simulink model "EBike_Braking"  (R2019b)
settings: Solver=VariableStepAuto  StartTime=0.0  StopTime=1000  MaxStep=0.01  RelTol=1e-3
values from neighbouring files (symbols this model uses):
  A_d = 0.4    [Thesis_Ebike.m]
  Abs = 1    [Thesis_Ebike.m]
  alpha_Conductor = 0.0040    (= 0.004)    [Thesis_Ebike.m]
  Alpha_Magnet = -0.0020    (= -0.002)    [Thesis_Ebike.m]
  Bm = ((Motor_torque_constant)*(17)/(1000*2*pi/60))    (= 0.121753531465)    [Thesis_Ebike.m]
  Braking_Pressure = 100    [Thesis_Ebike.m]
  C_d = 0.9    [Thesis_Ebike.m]
  capacity = 19.5    [Thesis_Ebike.m]
  Coefficient_of_Brake_friction = 0.9    [Thesis_Ebike.m]
  Crank_Length = 0.150    (= 0.15)    [Thesis_Ebike.m]
  Cyclist_weight = 85    [Thesis_Ebike.m]
  Dynamic_Friction_Coefficient = 0.0015    [Thesis_Ebike.m]
  Effective_Radius_of_Disc = 0.16    [Thesis_Ebike.m]
  F_Rider = 100    [Thesis_Ebike.m]
  g = 9.81    [Thesis_Ebike.m]
  Internal_Resistance = 95*10^-3    (= 0.095)    [Thesis_Ebike.m]
  Jm = 10.2 *10^-3    (= 0.0102)    [Thesis_Ebike.m]
  Kb = (51.7/(1000*2*pi/60))    (= 0.493698633471)    [Thesis_Ebike.m]
  L = 0.36*10^-3    (= 0.00036)    [Thesis_Ebike.m]
  Motor_resistance = 88*10^-2    (= 0.88)    [Thesis_Ebike.m]
  Motor_torque_constant = 0.75    [Thesis_Ebike.m]
  Polarization_Capacitance = 1*10^-7    (= 1e-07)    [Thesis_Ebike.m]
  Polarization_Resistance = 95*10^-3    (= 0.095)    [Thesis_Ebike.m]
  Ref_Temp = 25    [Thesis_Ebike.m]
  Rho_air = 1.225    [Thesis_Ebike.m]
  SOC_initial = 100    [Thesis_Ebike.m]
  Static_Friction_Coefficient = 0.0015    [Thesis_Ebike.m]
  Tire_mass = 0.25    [Thesis_Ebike.m]
  Trailer_mass = 50    [Thesis_Ebike.m]
  Vehicle_mass = 25    [Thesis_Ebike.m]
  Wheel_Inertia = 0.0225    [Thesis_Ebike.m]
  Wheel_mass = 0.25    [Thesis_Ebike.m]
  Wheel_Radius = 0.3    [Thesis_Ebike.m]
undefined symbols (not defined in the file or in its folder): sigbuilder_block, V
libraries: simulink x2
(part 2 of 3)

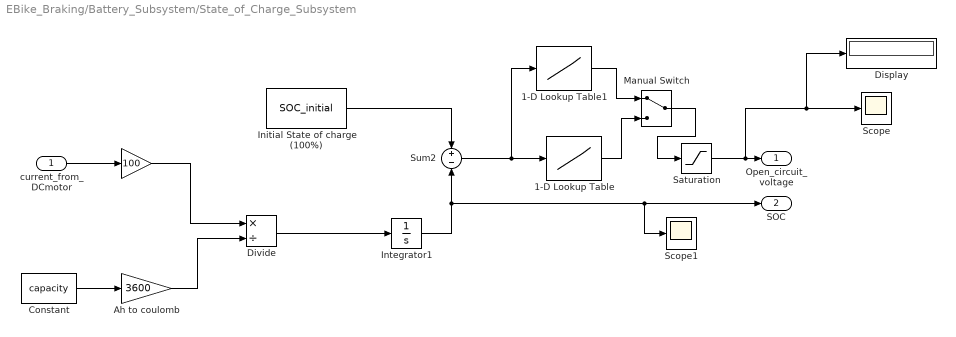
== system EBike_Braking/Battery_Subsystem/State_of_Charge_Subsystem  ==
  current_from_DCmotor : Inport
  " " : Gain  Gain=100
  1-D Lookup Table : Lookup_n-D  NumberOfTableDimensions=1  BreakpointsForDimension1=[10 12 15 20 30 45 60 75 85 95 100]  Table=|  InternalRulePriority=Speed  RndMeth=Simplest  InputSameDT=on
      | [2.75
      | 2.964
      | 3.233
      | 3.417
      | 3.65
      | 3.7
      | 3.789
      | 3.9269
      | 4.017
      | 4.147
      | 4.2
      | ]
  1-D Lookup Table1 : Lookup_n-D  NumberOfTableDimensions=1  BreakpointsForDimension1=|  Table=|  InternalRulePriority=Speed  RndMeth=Simplest  InputSameDT=on
      BreakpointsForDimension1=|
      | [-0.02
      | 0.08
      | 0.18
      | 0.28
      | 0.38
      | 0.48
      | 0.58
      | 0.68
      | 0.78
      | 0.88
      | 0.98
      | 1.08
      | 1.18
      | 1.28
      | 1.38
      | 1.48
      | 1.58
      | 1.68
      | 1.78
      | 1.88
      | 1.98
      | 2.08
      | 2.18
      | 2.28
      | 2.38
      | 2.48
      | 2.58
      | 2.68
      | 2.78
      | 2.88
      | 2.98
      | 3.08
      | 3.18
      | 3.28
      | 3.38
      | 3.48
      | 3.58
      | 3.68
      | 3.78
      | 3.88
      | 3.98
      | 4.08
      | 4.18
      | 4.28
      | 4.38
      | 4.48
      | 4.58
      | 4.68
      | 4.78
      | 4.88
      | 4.98
      | 5.08
      | 5.18
      | 5.28
      | 5.38
      | 5.48
      | 5.58
      | 5.68
      | 5.78
      | 5.88
      | 5.98
      | 6.08
      | 6.19
      | 6.29
      | 6.39
      | 6.49
      | 6.59
      | 6.69
      | 6.79
      | 6.89
      | 6.99
      | 7.09
      | 7.19
      | 7.29
      | 7.39
      | 7.49
      | 7.59
      | 7.69
      | 7.79
      | 7.89
      | 7.99
      | 8.09
      | 8.19
      | 8.29
      | 8.39
      | 8.49
      | 8.59
      | 8.69
      | 8.79
      | 8.89
      | 8.99
      | 9.09
      | 9.19
      | 9.29
      | 9.39
      | 9.49
      | 9.59
      | 9.69
      | 9.79
      | 9.89
      | 9.99
      | 10.09
      | 10.19
      | 10.29
      | 10.39
      | 10.49
      | 10.59
      | 10.69
      | 10.79
      | 10.89
      | 10.99
      | 11.09
      | 11.19
      | 11.29
      | 11.39
      | 11.49
      | 11.59
      | 11.69
      | 11.79
      | 11.89
      | 11.99
      | 12.09
      | 12.19
      | 12.29
      | 12.39
      | 12.49
      | 12.59
      | 12.69
      | 12.79
      | 12.89
      | 12.99
      | 13.09
      | 13.19
      | 13.29
      | 13.39
      | 13.49
      | 13.59
      | 13.69
      | 13.79
      | 13.89
      | 13.99
      | 14.09
      | 14.19
      | 14.29
      | 14.39
      | 14.49
      | 14.59
      | 14.69
      | 14.79
      | 14.89
      | 14.99
      | 15.09
      | 15.19
      | 15.29
      | 15.39
      | 15.49
      | 15.59
      | 15.69
      | 15.79
      | 15.89
      | 15.99
      | 16.09
      | 16.19
      | 16.29
      | 16.39
      | 16.49
      | 16.59
      | 16.69
      | 16.79
      | 16.89
      | 16.99
      | 17.09
      | 17.19
      | 17.29
      | 17.39
      | 17.49
      | 17.59
      | 17.69
      | 17.79
      | 17.89
      | 17.99
      | 18.09
      | 18.19
      | 18.29
      | 18.39
      | 18.49
      | 18.59
      | 18.69
      | 18.79
      | 18.89
      | 18.99
      | 19.09
      | 19.19
      | 19.29
      | 19.39
      | 19.49
      | 19.59
      | 19.69
      | 19.79
      | 19.89
      | 19.99
      | 20.09
      | 20.19
      | 20.29
      | 20.39
      | 20.49
      | 20.59
      | 20.69
      | 20.79
      | 20.89
      | 20.99
      | 21.09
      | 21.19
      | 21.29
      | 21.39
      | 21.49
      | 21.59
      | 21.69
      | 21.79
      | 21.89
      | 21.99
      | 22.09
      | 22.19
      | 22.29
      | 22.39
      | 22.49
      | 22.59
      | 22.69
      | 22.79
      | 22.89
      | 22.99
      | 23.09
      | 23.19
      | 23.29
      | 23.39
      | 23.49
      | 23.59
      | 23.69
      | 23.79
      | 23.89
      | 23.99
      | 24.09
      | 24.19
      | 24.29
      | 24.39
      | 24.49
      | 24.59
      | 24.69
      | 24.79
      | 24.89
      | 24.99
      | 25.09
      | 25.19
      | 25.29
      | 25.39
      | 25.49
      | 25.59
      | 25.69
      | 25.79
      | 25.89
      | 25.99
      | 26.09
      | 26.19
      | 26.29
      | 26.39
      | 26.49
      | 26.59
      | 26.69
      | 26.79
      | 26.89
      | 26.99
      | 27.09
      | 27.19
      | 27.29
      | 27.39
      | 27.49
      | 27.59
      | 27.69
      | 27.79
      | 27.89
      | 27.99
      | 28.09
      | 28.19
      | 28.29
      | 28.39
      | 28.49
      | 28.59
      | 28.69
      | 28.79
      | 28.89
      | 28.99
      | 29.09
      | 29.19
      | 29.29
      | 29.39
      | 29.49
      | 29.59
      | 29.69
      | 29.79
      | 29.89
      | 29.99
      | 30.09
      | 30.19
      | 30.29
      | 30.39
      | 30.49
      | 30.59
      | 30.69
      | 30.79
      | 30.89
      | 30.99
      | 31.09
      | 31.19
      | 31.29
      | 31.39
      | 31.49
      | 31.59
      | 31.69
      | 31.79
      | 31.89
      | 31.99
      | 32.09
      | 32.19
      | 32.29
      | 32.39
      | 32.49
      | 32.59
      | 32.69
      | 32.79
      | 32.89
      | 32.99
      | 33.09
      | 33.19
      | 33.29
      | 33.39
      | 33.49
      | 33.59
      | 33.69
      | 33.79
      | 33.89
      | 33.99
      | 34.09
      | 34.19
      | 34.29
      | 34.39
      | 34.49
      | 34.59
      | 34.69
      | 34.79
      | 34.89
      | 34.99
      | 35.09
      | 35.19
      | 35.29
      | 35.39
      | 35.49
      | 35.59
      | 35.69
      | 35.79
      | 35.89
      | 35.99
      | 36.09
      | 36.19
      | 36.29
      | 36.39
      | 36.49
      | 36.59
      | 36.69
      | 36.79
      | 36.89
      | 36.99
      | 37.09
      | 37.19
      | 37.29
      | 37.39
      | 37.49
      | 37.59
      | 37.69
      | 37.79
      | 37.89
      | 37.99
      | 38.09
      | 38.19
      | 38.29
      | 38.39
      | 38.49
      | 38.59
      | 38.69
      | 38.79
      | 38.89
      | 38.99
      | 39.09
      | 39.19
      | 39.29
      | 39.39
      | 39.49
      | 39.59
      | 39.69
      | 39.79
      | 39.89
      | 39.99
      | 40.09
      | 40.19
      | 40.29
      | 40.39
      | 40.49
      | 40.59
      | 40.69
      | 40.79
      | 40.89
      | 40.99
      | 41.09
      | 41.19
      | 41.29
      | 41.39
      | 41.49
      | 41.59
      | 41.69
      | 41.79
      | 41.89
      | 41.99
      | 42.09
      | 42.19
      | 42.29
      | 42.39
      | 42.49
      | 42.59
      | 42.69
      | 42.79
      | 42.89
      | 42.99
      | 43.09
      | 43.19
      | 43.29
      | 43.39
      | 43.49
      | 43.59
      | 43.69
      | 43.79
      | 43.89
      | 43.99
      | 44.09
      | 44.19
      | 44.29
      | 44.39
      | 44.49
      | 44.59
      | 44.69
      | 44.79
      | 44.89
      | 44.99
      | 45.09
      | 45.19
      | 45.29
      | 45.39
      | 45.49
      | 45.59
      | 45.69
      | 45.79
      | 45.89
      | 45.99
      | 46.09
      | 46.19
      | 46.29
      | 46.39
      | 46.49
      | 46.59
      | 46.69
      | 46.79
      | 46.89
      | 46.99
      | 47.09
      | 47.19
      | 47.29
      | 47.39
      | 47.49
      | 47.59
      | 47.69
      | 47.79
      | 47.89
      | 47.99
      | 48.09
      | 48.19
      | 48.29
      | 48.39
      | 48.49
      | 48.59
      | 48.69
      | 48.79
      | 48.89
      | 48.99
      | 49.09
      | 49.19
      | 49.29
      | 49.39
      | 49.49
      | 49.59
      | 49.69
      | 49.79
      | 49.89
      | 49.99
      | 50.09
      | 50.19
      | 50.29
      | 50.39
      | 50.49
      | 50.59
      | 50.69
      | 50.79
      | 50.89
      | 50.99
      | 51.09
      | 51.19
      | 51.29
      | 51.39
      | 51.49
      | 51.59
      | 51.69
      | 51.79
      | 51.89
      | 51.99
      | 52.09
      | 52.19
      | 52.29
      | 52.39
      | 52.49
      | 52.59
      | 52.69
      | 52.79
      | 52.89
      | 52.99
      | 53.09
      | 53.19
      | 53.29
      | 53.39
      | 53.49
      | 53.59
      | 53.69
      | 53.79
      | 53.89
      | 53.99
      | 54.09
      | 54.19
      | 54.29
      | 54.39
      | 54.49
      | 54.59
      | 54.69
      | 54.79
      | 54.89
      | 54.99
      | 55.09
      | 55.19
      | 55.29
      | 55.39
      | 55.49
      | 55.59
      | 55.69
      | 55.79
      | 55.89
      | 55.99
      | 56.09
      | 56.19
      | 56.29
      | 56.39
      | 56.49
      | 56.59
      | 56.69
      | 56.79
      | 56.89
      | 56.99
      | 57.09
      | 57.19
      | 57.29
      | 57.39
      | 57.49
      | 57.59
      | 57.69
      | 57.79
      | 57.89
      | 57.99
      | 58.09
      | 58.19
      | 58.29
      | 58.39
      | 58.49
      | 58.59
      | 58.69
      | 58.79
      | 58.89
      | 58.99
      | 59.09
      | 59.19
      | 59.29
      | 59.39
      | 59.49
      | 59.59
      | 59.69
      | 59.79
      | 59.89
      | 59.99
      | 60.09
      | 60.19
      | 60.29
      | 60.39
      | 60.49
      | 60.59
      | 60.69
      | 60.79
      | 60.89
      | 60.99
      | 61.09
      | 61.19
      | 61.29
      | 61.39
      | 61.49
      | 61.59
      | 61.69
      | 61.79
      | 61.89
      | 61.99
      | 62.09
      | 62.19
      | 62.29
      | 62.39
      | 62.49
      | 62.59
      | 62.69
      | 62.79
      | 62.89
      | 62.99
      | 63.09
      | 63.19
      | 63.29
      | 63.39
      | 63.49
      | 63.59
      | 63.69
      | 63.79
      | 63.89
      | 63.99
      | 64.09
      | 64.19
      | 64.29
      | 64.39
      | 64.49
      | 64.59
      | 64.69
      | 64.79
      | 64.89
      | 64.99
      | 65.09
      | 65.19
      | 65.29
      | 65.39
      | 65.49
      | 65.59
      | 65.69
      | 65.79
      | 65.89
      | 65.99
      | 66.09
      | 66.19
      | 66.29
      | 66.39
      | 66.49
      | 66.59
      | 66.69
      | 66.79
      | 66.89
      | 66.99
      | 67.09
      | 67.19
      | 67.29
      | 67.39
      | 67.49
      | 67.59
      | 67.69
      | 67.79
      | 67.89
      | 67.99
      | 68.09
      | 68.19
      | 68.29
      | 68.39
      | 68.49
      | 68.59
      | 68.69
      | 68.80
      | 68.90
      | 69.00
      | 69.10
      | 69.20
      | 69.30
      | 69.40
      | 69.50
      | 69.60
      | 69.70
      | 69.80
      | 69.90
      | 70.00
      | 70.10
      | 70.20
      | 70.30
      | 70.40
      | 70.50
      | 70.60
      | 70.70
      | 70.80
      | 70.90
      | 71.00
      | 71.10
      | 71.20
      | 71.30
      | 71.40
      | 71.50
      | 71.60
      | 71.70
      | 71.80
      | 71.90
      | 72.00
      | 72.10
      | 72.20
      | 72.30
      | 72.40
      | 72.50
      | 72.60
      | 72.70
      | 72.80
      | 72.90
      | 73.00
      | 73.10
      | 73.20
      | 73.30
      | 73.40
      | 73.50
      | 73.60
      | 73.70
      | 73.80
      | 73.90
      | 74.00
      | 74.10
      | 74.20
      | 74.30
      | 74.40
      | 74.50
      | 74.60
      | 74.70
      | 74.80
      | 74.90
      | 75.00
      | 75.10
      | 75.20
      | 75.30
      | 75.40
      | 75.50
      | 75.60
      | 75.70
      | 75.80
      | 75.90
      | 76.00
      | 76.10
      | 76.20
      | 76.30
      | 76.40
      | 76.50
      | 76.60
      | 76.70
      | 76.80
      | 76.90
      | 77.00
      | 77.10
      | 77.20
      | 77.30
      | 77.40
      | 77.50
      | 77.60
      | 77.70
      | 77.80
      | 77.90
      | 78.00
      | 78.10
      | 78.20
      | 78.30
      | 78.40
      | 78.50
      | 78.60
      | 78.70
      | 78.80
      | 78.90
      | 79.00
      | 79.10
      | 79.20
      | 79.30
      | 79.40
      | 79.50
      | 79.60
      | 79.70
      | 79.80
      | 79.90
      | 80.00
      | 80.10
      | 80.20
      | 80.30
      | 80.40
      | 80.50
      | 80.60
      | 80.70
      | 80.80
      | 80.90
      | 81.00
      | 81.10
      | 81.20
      | 81.30
      | 81.40
      | 81.50
      | 81.60
      | 81.70
      | 81.80
      | 81.90
      | 82.00
      | 82.10
      | 82.20
      | 82.30
      | 82.40
      | 82.50
      | 82.60
      | 82.70
      | 82.80
      | 82.90
      | 83.00
      | 83.10
      | 83.20
      | 83.30
      | 83.40
      | 83.50
      | 83.60
      | 83.70
      | 83.80
      | 83.90
      | 84.00
      | 84.10
      | 84.20
      | 84.30
      | 84.40
      | 84.50
      | 84.60
      | 84.70
      | 84.80
      | 84.90
      | 85.00
      | 85.10
      | 85.20
      | 85.30
      | 85.40
      | 85.50
      | 85.60
      | 85.70
      | 85.80
      | 85.90
      | 86.00
      | 86.10
      | 86.20
      | 86.30
      | 86.40
      | 86.50
      | 86.60
      | 86.70
      | 86.80
      | 86.90
      | 87.00
      | 87.10
      | 87.20
      | 87.30
      | 87.40
      | 87.50
      | 87.60
      | 87.70
      | 87.80
      | 87.90
      | 88.00
      | 88.10
      | 88.20
      | 88.30
      | 88.40
      | 88.50
      | 88.60
      | 88.70
      | 88.80
      | 88.90
      | 89.00
      | 89.10
      | 89.20
      | 89.30
      | 89.40
      | 89.50
      | 89.60
      | 89.70
      | 89.80
      | 89.90
      | 90.00
      | 90.10
      | 90.20
      | 90.30
      | 90.40
      | 90.50
      | 90.60
      | 90.70
      | 90.80
      | 90.90
      | 91.00
      | 91.10
      | 91.20
      | 91.30
      | 91.40
      | 91.50
      | 91.60
      | 91.70
      | 91.80
      | 91.90
      | 92.00
      | 92.10
      | 92.20
      | 92.30
      | 92.40
      | 92.50
      | 92.60
      | 92.70
      | 92.80
      | 92.90
      | 93.00
      | 93.10
      | 93.20
      | 93.30
      | 93.40
      | 93.50
      | 93.60
      | 93.70
      | 93.80
      | 93.90
      | 94.00
      | 94.10
      | 94.20
      | 94.30
      | 94.40
      | 94.50
      | 94.60
      | 94.70
      | 94.80
      | 94.90
      | 95.00
      | 95.10
      | 95.20
      | 95.30
      | 95.40
      | 95.50
      | 95.60
      | 95.70
      | 95.80
      | 95.90
      | 96.00
      | 96.10
      | 96.20
      | 96.30
      | 96.40
      | 96.50
      | 96.60
      | 96.70
      | 96.80
      | 96.90
      | 97.00
      | 97.10
      | 97.20
      | 97.30
      | 97.40
      | 97.50
      | 97.60
      | 97.70
      | 97.80
      | 97.90
      | 98.00
      | 98.10
      | 98.20
      | 98.30
      | 98.40
      | 98.50
      | 98.60
      | 98.70
      | 98.80
      | 98.90
      | 99.00
      | 99.10
      | 99.20
      | 99.30
      | 99.40
      | 99.50
      | 99.60
      | 99.70
      | 99.80
      | 99.90
      | ]
      Table=|
      | [26.9
      | 27.2
      | 27.4
      | 27.6
      | 27.9
      | 28.1
      | 28.3
      | 28.5
      | 28.7
      | 28.9
      | 29.1
      | 29.3
      | 29.5
      | 29.6
      | 29.8
      | 30
      | 30.1
      | 30.3
      | 30.4
      | 30.6
      | 30.7
      | 30.8
      | 31
      | 31.1
      | 31.2
      | 31.3
      | 31.4
      | 31.5
      | 31.6
      | 31.7
      | 31.8
      | 31.9
      | 32
      | 32.1
      | 32.2
      | 32.2
      | 32.3
      | 32.4
      | 32.4
      | 32.5
      | 32.6
      | 32.6
      | 32.7
      | 32.7
      | 32.8
      | 32.8
      | 32.9
      | 32.9
      | 32.9
      | 33
      | 33
      | 33.1
      | 33.1
      | 33.1
      | 33.1
      | 33.2
      | 33.2
      | 33.2
      | 33.2
      | 33.3
      | 33.3
      | 33.3
      | 33.3
      | 33.3
      | 33.3
      | 33.4
      | 33.4
      | 33.4
      | 33.4
      | 33.4
      | 33.4
      | 33.4
      | 33.5
      | 33.5
      | 33.5
      | 33.5
      | 33.5
      | 33.5
      | 33.5
      | 33.6
      | 33.6
      | 33.6
      | 33.6
      | 33.6
      | 33.6
      | 33.6
      | 33.6
      | 33.7
      | 33.7
      | 33.7
      | 33.7
      | 33.7
      | 33.7
      | 33.7
      | 33.8
      | 33.8
      | 33.8
      | 33.8
      | 33.8
      | 33.8
      | 33.8
      | 33.8
      | 33.9
      | 33.9
      | 33.9
      | 33.9
      | 33.9
      | 33.9
      | 33.9
      | 33.9
      | 33.9
      | 34
      | 34
      | 34
      | 34
      | 34
      | 34
      | 34
      | 34
      | 34
      | 34
      | 34.1
      | 34.1
      | 34.1
      | 34.1
      | 34.1
      | 34.1
      | 34.1
      | 34.1
      | 34.1
      | 34.1
      | 34.1
      | 34.2
      | 34.2
      | 34.2
      | 34.2
      | 34.2
      | 34.2
      | 34.2
      | 34.2
      | 34.2
      | 34.2
      | 34.2
      | 34.2
      | 34.3
      | 34.3
      | 34.3
      | 34.3
      | 34.3
      | 34.3
      | 34.3
      | 34.3
      | 34.3
      | 34.3
      | 34.3
      | 34.3
      | 34.3
      | 34.4
      | 34.4
      | 34.4
      | 34.4
      | 34.4
      | 34.4
      | 34.4
      | 34.4
      | 34.4
      | 34.4
      | 34.4
      | 34.4
      | 34.4
      | 34.4
      | 34.4
      | 34.5
      | 34.5
      | 34.5
      | 34.5
      | 34.5
      | 34.5
      | 34.5
      | 34.5
      | 34.5
      | 34.5
      | 34.5
      | 34.5
      | 34.5
      | 34.5
      | 34.5
      | 34.5
      | 34.6
      | 34.6
      | 34.6
      | 34.6
      | 34.6
      | 34.6
      | 34.6
      | 34.6
      | 34.6
      | 34.6
      | 34.6
      | 34.6
      | 34.6
      | 34.6
      | 34.6
      | 34.6
      | 34.6
      | 34.6
      | 34.6
      | 34.6
      | 34.7
      | 34.7
      | 34.7
      | 34.7
      | 34.7
      | 34.7
      | 34.7
      | 34.7
      | 34.7
      | 34.7
      | 34.7
      | 34.7
      | 34.7
      | 34.7
      | 34.7
      | 34.7
      | 34.7
      | 34.7
      | 34.7
      | 34.7
      | 34.7
      | 34.7
      | 34.8
      | 34.8
      | 34.8
      | 34.8
      | 34.8
      | 34.8
      | 34.8
      | 34.8
      | 34.8
      | 34.8
      | 34.8
      | 34.8
      | 34.8
      | 34.8
      | 34.8
      | 34.8
      | 34.8
      | 34.8
      | 34.8
      | 34.8
      | 34.8
      | 34.8
      | 34.8
      | 34.8
      | 34.8
      | 34.9
      | 34.9
      | 34.9
      | 34.9
      | 34.9
      | 34.9
      | 34.9
      | 34.9
      | 34.9
      | 34.9
      | 34.9
      | 34.9
      | 34.9
      | 34.9
      | 34.9
      | 34.9
      | 34.9
      | 34.9
      | 34.9
      | 34.9
      | 34.9
      | 34.9
      | 34.9
      | 34.9
      | 34.9
      | 34.9
      | 34.9
      | 35
      | 35
      | 35
      | 35
      | 35
      | 35
      | 35
      | 35
      | 35
      | 35
      | 35
      | 35
      | 35
      | 35
      | 35
      | 35
      | 35
      | 35
      | 35
      | 35
      | 35
      | 35
      | 35
      | 35
      | 35
      | 35
      | 35
      | 35
      | 35.1
      | 35.1
      | 35.1
      | 35.1
      | 35.1
      | 35.1
      | 35.1
      | 35.1
      | 35.1
      | 35.1
      | 35.1
      | 35.1
      | 35.1
      | 35.1
      | 35.1
      | 35.1
      | 35.1
      | 35.1
      | 35.1
      | 35.1
      | 35.1
      | 35.1
      | 35.1
      | 35.1
      | 35.1
      | 35.1
      | 35.1
      | 35.1
      | 35.1
      | 35.1
      | 35.1
      | 35.2
      | 35.2
      | 35.2
      | 35.2
      | 35.2
      | 35.2
      | 35.2
      | 35.2
      | 35.2
      | 35.2
      | 35.2
      | 35.2
      | 35.2
      | 35.2
      | 35.2
      | 35.2
      | 35.2
      | 35.2
      | 35.2
      | 35.2
      | 35.2
      | 35.2
      | 35.2
      | 35.2
      | 35.2
      | 35.2
      | 35.2
      | 35.2
      | 35.2
      | 35.2
      | 35.3
      | 35.3
      | 35.3
      | 35.3
      | 35.3
      | 35.3
      | 35.3
      | 35.3
      | 35.3
      | 35.3
      | 35.3
      | 35.3
      | 35.3
      | 35.3
      | 35.3
      | 35.3
      | 35.3
      | 35.3
      | 35.3
      | 35.3
      | 35.3
      | 35.3
      | 35.3
      | 35.3
      | 35.3
      | 35.3
      | 35.3
      | 35.3
      | 35.4
      | 35.4
      | 35.4
      | 35.4
      | 35.4
      | 35.4
      | 35.4
      | 35.4
      | 35.4
      | 35.4
      | 35.4
      | 35.4
      | 35.4
      | 35.4
      | 35.4
      | 35.4
      | 35.4
      | 35.4
      | 35.4
      | 35.4
      | 35.4
      | 35.4
      | 35.4
      | 35.4
      | 35.4
      | 35.4
      | 35.5
      | 35.5
      | 35.5
      | 35.5
      | 35.5
      | 35.5
      | 35.5
      | 35.5
      | 35.5
      | 35.5
      | 35.5
      | 35.5
      | 35.5
      | 35.5
      | 35.5
      | 35.5
      | 35.5
      | 35.5
      | 35.5
      | 35.5
      | 35.5
      | 35.5
      | 35.5
      | 35.6
      | 35.6
      | 35.6
      | 35.6
      | 35.6
      | 35.6
      | 35.6
      | 35.6
      | 35.6
      | 35.6
      | 35.6
      | 35.6
      | 35.6
      | 35.6
      | 35.6
      | 35.6
      | 35.6
      | 35.6
      | 35.6
      | 35.6
      | 35.6
      | 35.6
      | 35.6
      | 35.7
      | 35.7
      | 35.7
      | 35.7
      | 35.7
      | 35.7
      | 35.7
      | 35.7
      | 35.7
      | 35.7
      | 35.7
      | 35.7
      | 35.7
      | 35.7
      | 35.7
      | 35.7
      | 35.7
      | 35.7
      | 35.7
      | 35.7
      | 35.8
      | 35.8
      | 35.8
      | 35.8
      | 35.8
      | 35.8
      | 35.8
      | 35.8
      | 35.8
      | 35.8
      | 35.8
      | 35.8
      | 35.8
      | 35.8
      | 35.8
      | 35.8
      | 35.8
      | 35.8
      | 35.8
      | 35.9
      | 35.9
      | 35.9
      | 35.9
      | 35.9
      | 35.9
      | 35.9
      | 35.9
      | 35.9
      | 35.9
      | 35.9
      | 35.9
      | 35.9
      | 35.9
      | 35.9
      | 35.9
      | 35.9
      | 35.9
      | 36
      | 36
      | 36
      | 36
      | 36
      | 36
      | 36
      | 36
      | 36
      | 36
      | 36
      | 36
      | 36
      | 36
      | 36
      | 36
      | 36
      | 36.1
      | 36.1
      | 36.1
      | 36.1
      | 36.1
      | 36.1
      | 36.1
      | 36.1
      | 36.1
      | 36.1
      | 36.1
      | 36.1
      | 36.1
      | 36.1
      | 36.1
      | 36.1
      | 36.2
      | 36.2
      | 36.2
      | 36.2
      | 36.2
      | 36.2
      | 36.2
      | 36.2
      | 36.2
      | 36.2
      | 36.2
      | 36.2
      | 36.2
      | 36.2
      | 36.3
      | 36.3
      | 36.3
      | 36.3
      | 36.3
      | 36.3
      | 36.3
      | 36.3
      | 36.3
      | 36.3
      | 36.3
      | 36.3
      | 36.3
      | 36.4
      | 36.4
      | 36.4
      | 36.4
      | 36.4
      | 36.4
      | 36.4
      | 36.4
      | 36.4
      | 36.4
      | 36.4
      | 36.4
      | 36.4
      | 36.5
      | 36.5
      | 36.5
      | 36.5
      | 36.5
      | 36.5
      | 36.5
      | 36.5
      | 36.5
      | 36.5
      | 36.5
      | 36.5
      | 36.6
      | 36.6
      | 36.6
      | 36.6
      | 36.6
      | 36.6
      | 36.6
      | 36.6
      | 36.6
      | 36.6
      | 36.6
      | 36.6
      | 36.7
      | 36.7
      | 36.7
      | 36.7
      | 36.7
      | 36.7
      | 36.7
      | 36.7
      | 36.7
      | 36.7
      | 36.7
      | 36.8
      | 36.8
      | 36.8
      | 36.8
      | 36.8
      | 36.8
      | 36.8
      | 36.8
      | 36.8
      | 36.8
      | 36.9
      | 36.9
      | 36.9
      | 36.9
      | 36.9
      | 36.9
      | 36.9
      | 36.9
      | 36.9
      | 36.9
      | 36.9
      | 37
      | 37
      | 37
      | 37
      | 37
      | 37
      | 37
      | 37
      | 37
      | 37
      | 37.1
      | 37.1
      | 37.1
      | 37.1
      | 37.1
      | 37.1
      | 37.1
      | 37.1
      | 37.1
      | 37.1
      | 37.2
      | 37.2
      | 37.2
      | 37.2
      | 37.2
      | 37.2
      | 37.2
      | 37.2
      | 37.2
      | 37.2
      | 37.3
      | 37.3
      | 37.3
      | 37.3
      | 37.3
      | 37.3
      | 37.3
      | 37.3
      | 37.3
      | 37.4
      | 37.4
      | 37.4
      | 37.4
      | 37.4
      | 37.4
      | 37.4
      | 37.4
      | 37.4
      | 37.4
      | 37.5
      | 37.5
      | 37.5
      | 37.5
      | 37.5
      | 37.5
      | 37.5
      | 37.5
      | 37.5
      | 37.6
      | 37.6
      | 37.6
      | 37.6
      | 37.6
      | 37.6
      | 37.6
      | 37.6
      | 37.6
      | 37.7
      | 37.7
      | 37.7
      | 37.7
      | 37.7
      | 37.7
      | 37.7
      | 37.7
      | 37.7
      | 37.8
      | 37.8
      | 37.8
      | 37.8
      | 37.8
      | 37.8
      | 37.8
      | 37.8
      | 37.8
      | 37.8
      | 37.9
      | 37.9
      | 37.9
      | 37.9
      | 37.9
      | 37.9
      | 37.9
      | 37.9
      | 37.9
      | 38
      | 38
      | 38
      | 38
      | 38
      | 38
      | 38
      | 38
      | 38
      | 38
      | 38.1
      | 38.1
      | 38.1
      | 38.1
      | 38.1
      | 38.1
      | 38.1
      | 38.1
      | 38.1
      | 38.2
      | 38.2
      | 38.2
      | 38.2
      | 38.2
      | 38.2
      | 38.2
      | 38.2
      | 38.3
      | 38.3
      | 38.3
      | 38.3
      | 38.3
      | 38.3
      | 38.3
      | 38.3
      | 38.3
      | 38.4
      | 38.4
      | 38.4
      | 38.4
      | 38.4
      | 38.4
      | 38.4
      | 38.4
      | 38.5
      | 38.5
      | 38.5
      | 38.5
      | 38.5
      | 38.5
      | 38.5
      | 38.5
      | 38.5
      | 38.6
      | 38.6
      | 38.6
      | 38.6
      | 38.6
      | 38.6
      | 38.6
      | 38.6
      | 38.7
      | 38.7
      | 38.7
      | 38.7
      | 38.7
      | 38.7
      | 38.7
      | 38.7
      | 38.7
      | 38.8
      | 38.8
      | 38.8
      | 38.8
      | 38.8
      | 38.8
      | 38.8
      | 38.8
      | 38.9
      | 38.9
      | 38.9
      | 38.9
      | 38.9
      | 38.9
      | 38.9
      | 38.9
      | 39
      | 39
      | 39
      | 39
      | 39
      | 39
      | 39
      | 39
      | 39.1
      | 39.1
      | 39.1
      | 39.1
      | 39.1
      | 39.1
      | 39.1
      | 39.1
      | 39.2
      | 39.2
      | 39.2
      | 39.2
      | 39.2
      | 39.2
      | 39.2
      | 39.2
      | 39.3
      | 39.3
      | 39.3
      | 39.3
      | 39.3
      | 39.3
      | 39.3
      | 39.3
      | 39.4
      | 39.4
      | 39.4
      | 39.4
      | 39.4
      | 39.4
      | 39.4
      | 39.4
      | 39.5
      | 39.5
      | 39.5
      | 39.5
      | 39.5
      | 39.5
      | 39.5
      | 39.5
      | 39.6
      | 39.6
      | 39.6
      | 39.6
      | 39.6
      | 39.6
      | 39.6
      | 39.6
      | 39.7
      | 39.7
      | 39.7
      | 39.7
      | 39.7
      | 39.7
      | 39.7
      | 39.7
      | 39.8
      | 39.8
      | 39.8
      | 39.8
      | 39.8
      | 39.8
      | 39.8
      | 39.9
      | 39.9
      | 39.9
      | 39.9
      | 39.9
      | 39.9
      | 39.9
      | 39.9
      | 40
      | 40
      | 40
      | 40
      | 40
      | 40
      | 40
      | 40.1
      | 40.1
      | 40.1
      | 40.1
      | 40.1
      | 40.1
      | 40.1
      | 40.1
      | 40.2
      | 40.2
      | 40.2
      | 40.2
      | 40.2
      | 40.2
      | 40.2
      | 40.3
      | 40.3
      | 40.3
      | 40.3
      | 40.3
      | 40.3
      | 40.3
      | 40.4
      | 40.4
      | 40.4
      | 40.4
      | 40.4
      | 40.4
      | 40.4
      | 40.5
      | 40.5
      | 40.5
      | 40.5
      | 40.5
      | 40.5
      | 40.5
      | 40.6
      | 40.6
      | 40.6
      | 40.6
      | 40.6
      | 40.6
      | 40.6
      | 40.7
      | 40.7
      | 40.7
      | 40.7
      | 40.7
      | 40.7
      | 40.8
      | 40.8
      | 40.8
      | 40.8
      | 40.8
      | 40.8
      | 40.8
      | 40.9
      | 40.9
      | 40.9
      | 40.9
      | 40.9
      | 40.9
      | 41
      | 41
      | 41
      | 41
      | 41
      | 41
      | 41
      | 41.1
      | 41.1
      | 41.1
      | 41.1
      | 41.1
      | 41.1
      | 41.2
      | ]
  Ah to coulomb : Gain  Gain=3600
  Constant : Constant  Value=capacity  SampleTime=-1
  Display : Display
  Divide : Product  Inputs=*/
  Initial State of charge (100%) : Constant  Value=SOC_initial  SampleTime=-1
  Integrator1 : Integrator  UpperSaturationLimit=100  LowerSaturationLimit=0
  Manual Switch : ManualSwitch
  Saturation : Saturate  UpperLimit=inf  LowerLimit=0
  Scope : Scope
  Scope1 : Scope
  Sum2 : Sum  Inputs=+|-
  Open_circuit_voltage : Outport  VectorParamsAs1DForOutWhenUnconnected=off
  SOC : Outport  Port=2  VectorParamsAs1DForOutWhenUnconnected=off
  wires:
  Integrator1/1 -> Scope1/1, SOC/1, Sum2/2
  Initial State of charge (100%)/1 -> Sum2/1
  Divide/1 -> Integrator1/1
  Saturation/1 -> Display/1, Scope/1, Open_circuit_voltage/1
  Sum2/1 -> 1-D Lookup Table/1, 1-D Lookup Table1/1
  Ah to coulomb/1 -> Divide/2
  current_from_DCmotor/1 -> " "/1
  Constant/1 -> Ah to coulomb/1
  " "/1 -> Divide/1
  1-D Lookup Table1/1 -> Manual Switch/1
  Manual Switch/1 -> Saturation/1
  1-D Lookup Table/1 -> Manual Switch/2

== system EBike_Braking/Bike_Mechanics_subsystem/Aerodynamic_Drag_subsystem ==
  Vehicle Speed (V) : Inport
  "Wind Speed (V_w) " : Inport  Port=2
  . : Constant  Value=1/2
  Air_density : Constant  Value=Rho_air
  Cross sectional area/Reference area : Constant  Value=A_d
  Drag Coeffient : Constant  Value=C_d
  Drag_force_scope : Scope
  Math Function1 : Math  Operator=square  SaturateOnIntegerOverflow=on
  Product : Product  Inputs=5
  Sum : Sum  Inputs=+-
  "Drag_Force " : Outport  VectorParamsAs1DForOutWhenUnconnected=off
  wires:
  Product/1 -> Drag_force_scope/1, "Drag_Force "/1
  ./1 -> Product/1
  Air_density/1 -> Product/2
  Drag Coeffient/1 -> Product/3
  Cross sectional area/Reference area/1 -> Product/4
  Math Function1/1 -> Product/5
  "Wind Speed (V_w) "/1 -> Sum/2
  Vehicle Speed (V)/1 -> Sum/1
  Sum/1 -> Math Function1/1

== system EBike_Braking/Bike_Mechanics_subsystem/Gradient_Resistance_subsystem ==
  Angle_of_slope : Inport
  Acceleration due to Gravity (g) m/s^2 : Constant  Value=g  SampleTime=-1
  Cos : Trigonometry
  Cyclist_weight (M) in Kg : Constant  Value=Cyclist_weight  SampleTime=-1
  Display : Display
  Gradient_resistance_scope : Scope
  Product : Product  Inputs=3
  Scope : Scope
  Sum2 : Sum
  Vehicle_mass (M) in Kg : Constant  Value=Vehicle_mass  SampleTime=-1
  Gradient_resistance : Outport  VectorParamsAs1DForOutWhenUnconnected=off
  wires:
  Product/1 -> Gradient_resistance_scope/1, Gradient_resistance/1
  Angle_of_slope/1 -> Cos/1
  Acceleration due to Gravity (g) m/s^2/1 -> Product/2
  Cos/1 -> Scope/1, Display/1, Product/3
  Sum2/1 -> Product/1
  Cyclist_weight (M) in Kg/1 -> Sum2/1
  Vehicle_mass (M) in Kg/1 -> Sum2/2

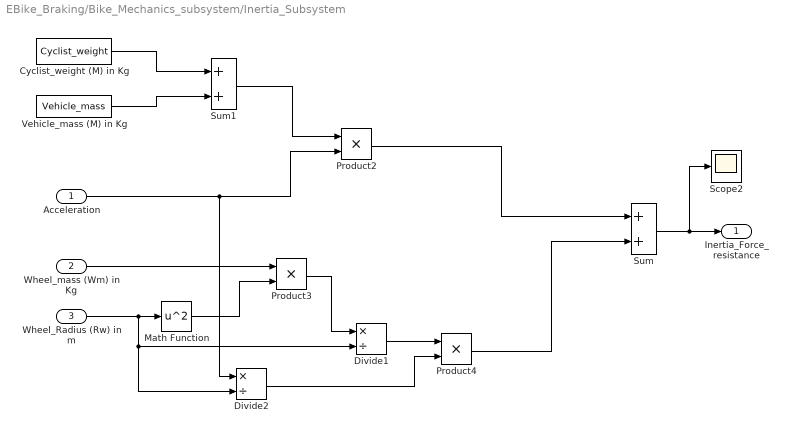
== system EBike_Braking/Bike_Mechanics_subsystem/Inertia_Subsystem ==
  Acceleration : Inport
  Wheel_mass (Wm) in Kg : Inport  Port=2
  Wheel_Radius (Rw) in m : Inport  Port=3
  Cyclist_weight (M) in Kg : Constant  Value=Cyclist_weight  SampleTime=-1
  Divide1 : Product  Inputs=*/
  Divide2 : Product  Inputs=*/
  Math Function : Math  Operator=square  SaturateOnIntegerOverflow=on
  Product2 : Product
  Product3 : Product
  Product4 : Product
  Scope2 : Scope
  Sum : Sum
  Sum1 : Sum
  Vehicle_mass (M) in Kg : Constant  Value=Vehicle_mass  SampleTime=-1
  Inertia_Force_resistance : Outport
  wires:
  Wheel_Radius (Rw) in m/1 -> Divide2/2, Divide1/2, Math Function/1
  Wheel_mass (Wm) in Kg/1 -> Product3/1
  Math Function/1 -> Product3/2
  Cyclist_weight (M) in Kg/1 -> Sum1/1
  Vehicle_mass (M) in Kg/1 -> Sum1/2
  Acceleration/1 -> Divide2/1, Product2/2
  Sum1/1 -> Product2/1
  Product3/1 -> Divide1/1
  Divide1/1 -> Product4/1
  Divide2/1 -> Product4/2
  Sum/1 -> Scope2/1, Inertia_Force_resistance/1
  Product2/1 -> Sum/1
  Product4/1 -> Sum/2

== system EBike_Braking/Bike_Mechanics_subsystem/Inertia_Subsystem1 ==
  Acceleration : Inport
  Gain : Gain
  Product2 : Product
  Scope2 : Scope
  Vehicle_mass (M) in Kg : Constant  Value=Trailer_mass  SampleTime=-1
  Trailer_force : Outport
  wires:
  Product2/1 -> Gain/1
  Vehicle_mass (M) in Kg/1 -> Product2/1
  Acceleration/1 -> Product2/2
  Gain/1 -> Scope2/1, Trailer_force/1

== system EBike_Braking/Bike_Mechanics_subsystem/Pedallic_torque_subsystem ==
  Torque : Inport
  Gear_ratio : Inport  Port=2
  Divide : Product  Inputs=*/
  Divide1 : Product  Inputs=*/
  Scope : Scope
  Scope1 : Scope
  Scope2 : Scope
  "Wheel_radius (Rw) " : Constant  Value=Wheel_Radius  SampleTime=-1
  Drive_Force : Outport  VectorParamsAs1DForOutWhenUnconnected=off
  wires:
  Gear_ratio/1 -> Divide1/2
  Divide1/1 -> Scope/1, Divide/1
  "Wheel_radius (Rw) "/1 -> Divide/2
  Divide/1 -> Scope2/1, Drive_Force/1
  Torque/1 -> Divide1/1, Scope1/1

== system EBike_Braking/Bike_Mechanics_subsystem/Rolling_Resistance_subsystem ==
  Angle_of_slope : Inport
  Acceleration_due_to_Gravity (g) m/s^2 : Constant  Value=g  SampleTime=-1
  Cos : Trigonometry  Operator=cos
  Cyclist_weight (M) in Kg : Constant  Value=Cyclist_weight  SampleTime=-1
  Dynamic_Friction_Coefficient : Constant  Value=Dynamic_Friction_Coefficient  SampleTime=-1
  Product : Product  Inputs=4
  Rolling_resistance_scope : Scope
  Static_Friction_Coefficient : Constant  Value=Static_Friction_Coefficient  SampleTime=-1
  Sum : Sum  Inputs=+|+
  Sum2 : Sum
  Vehicle_mass (M) in Kg : Constant  Value=Vehicle_mass  SampleTime=-1
  Rolling_resistance : Outport  VectorParamsAs1DForOutWhenUnconnected=off
  wires:
  Acceleration_due_to_Gravity (g) m/s^2/1 -> Product/3
  Product/1 -> Rolling_resistance/1, Rolling_resistance_scope/1
  Cos/1 -> Product/4
  Angle_of_slope/1 -> Cos/1
  Static_Friction_Coefficient/1 -> Sum/1
  Dynamic_Friction_Coefficient/1 -> Sum/2
  Sum/1 -> Product/1
  Sum2/1 -> Product/2
  Cyclist_weight (M) in Kg/1 -> Sum2/1
  Vehicle_mass (M) in Kg/1 -> Sum2/2

== system EBike_Braking/Bike_Mechanics_subsystem/Subsystem2 ==
  Slope % : Inport
  Constant : Constant  Value=pi  SampleTime=-1
  Constant1 : Constant  Value=180
  Divide : Product  Inputs=*/
  Gain : Gain  Gain=1/1
  Product : Product
  Trigonometric Function : Trigonometry  Operator=atan
  alpha : Outport  VectorParamsAs1DForOutWhenUnconnected=off
  wires:
  Gain/1 -> Trigonometric Function/1
  Slope %/1 -> Gain/1
  Trigonometric Function/1 -> Product/1
  Product/1 -> alpha/1
  Constant/1 -> Divide/1
  Constant1/1 -> Divide/2
  Divide/1 -> Product/2

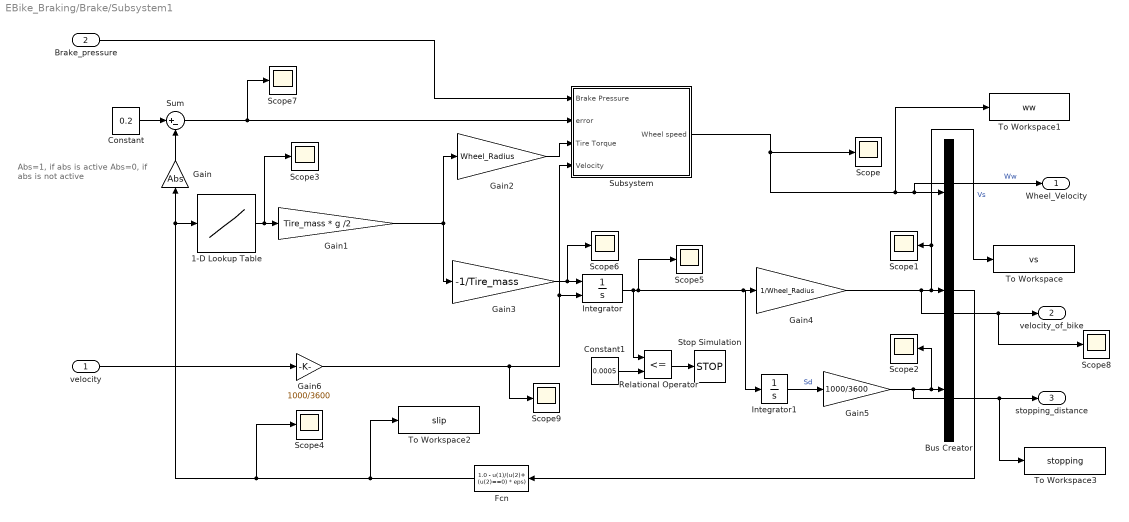
== system EBike_Braking/Brake/Subsystem1 ==
  note: Abs=1, if abs is active
      | Abs=0, if abs is not active
  velocity : Inport
  Brake_pressure : Inport  Port=2
  1-D Lookup Table : Lookup_n-D  NumberOfTableDimensions=1  BreakpointsForDimension1="[0\t0.0500000000000000\t0.100000000000000\t0.150000000000000\t0.200000000000000\t0.250000000000000\t0.300000000000000\t0.350000000000000\t0.400000000000000\t0.450000000000000\t0.500000000000000\t0.550000000000000\t0.600000000000000\t0.650000000000000\t0.700000000000000\t0.750000000000000\t0.800000000000000\t0.850000000000000\t0.900000000000000\t0.950000000000000\t1]"  Table="[0\t0.400000000000000\t0.800000000000000\t0.970000000000000\t1\t0.980000000000000\t0.960000000000000\t0.940000000000000\t0.920000000000000\t0.900000000000000\t0.880000000000000\t0.855000000000000\t0.830000000000000\t0.810000000000000\t0.790000000000000\t0.770000000000000\t0.750000000000000\t0.730000000000000\t0.720000000000000\t0.710000000000000\t0.700000000000000]"  InternalRulePriority=Speed  RndMeth=Simplest  InputSameDT=on
  Bus Creator : BusCreator  Inputs=3
  Constant : Constant  Value=0.2
  Constant1 : Constant  Value=0.0005
  Fcn : Fcn  Expr=1.0 - u(1)/(u(2)+ (u(2)==0) * eps)
  Gain : Gain  Gain=Abs
  Gain1 : Gain  Gain=Tire_mass * g /2
  Gain2 : Gain  Gain=Wheel_Radius
  Gain3 : Gain  Gain=-1/Tire_mass
  Gain4 : Gain  Gain=1/Wheel_Radius
  Gain5 : Gain  Gain=1000/3600
  Gain6 : Gain  Gain=1000/3600
  Integrator : Integrator  InitialConditionSource=external  InitialCondition=V  LimitOutput=on  UpperSaturationLimit=1000  LowerSaturationLimit=0  ZeroCross=off
  Integrator1 : Integrator
  Relational Operator : RelationalOperator  Operator=<=  OutDataTypeStr=boolean  RndMeth=Simplest
  Scope{,1..9} (10 alike) : Scope
  Stop Simulation : Stop
  Subsystem : Subsystem
  Sum : Sum  Inputs=|+-
  To Workspace : ToWorkspace  VariableName=vs  SaveFormat=Timeseries  SampleTime=-1
  To Workspace1 : ToWorkspace  VariableName=ww  SaveFormat=Timeseries  SampleTime=-1
  To Workspace2 : ToWorkspace  VariableName=slip  SaveFormat=Timeseries  SampleTime=-1
  To Workspace3 : ToWorkspace  VariableName=stopping  SaveFormat=Timeseries  SampleTime=-1
  Wheel_Velocity : Outport
  velocity_of_bike : Outport  Port=2
  stopping_distance : Outport  Port=3
  wires:
  Subsystem/1("Wheel speed ") -> Scope/1, To Workspace1/1, Wheel_Velocity/1, Bus Creator/1  "Ww"
  Integrator1/1 -> Gain5/1  "Sd"
  Sum/1 -> Subsystem/2("error "), Scope7/1
  Gain1/1 -> Gain3/1, Gain2/1
  Gain2/1 -> Subsystem/3(Tire Torque)
  Gain/1 -> Sum/2
  1-D Lookup Table/1 -> Scope3/1, Gain1/1
  Gain3/1 -> Scope6/1, Integrator/1
  Constant/1 -> Sum/1
  Gain4/1 -> To Workspace/1, Scope1/1, Bus Creator/2, Scope8/1, velocity_of_bike/1  "Vs"
  Fcn/1 -> To Workspace2/1, Scope4/1, 1-D Lookup Table/1, Gain/1
  Bus Creator/1 -> Fcn/1
  Constant1/1 -> Relational Operator/2
  Relational Operator/1 -> Stop Simulation/1
  Integrator/1 -> Integrator1/1, Gain4/1, Scope5/1, Relational Operator/1
  Gain5/1 -> To Workspace3/1, stopping_distance/1, Scope2/1, Bus Creator/3
  Gain6/1 -> Scope9/1, Subsystem/4(Velocity), Integrator/2
  Brake_pressure/1 -> Subsystem/1(Brake Pressure)
  velocity/1 -> Gain6/1

== system EBike_Braking/Controller/If Action Subsystem1 ==
  In1 : Inport
  Action Port : ActionPort  ActionPortLabel=if(u1<26)
  Gain : Gain
  Out1 : Outport
  wires:
  In1/1 -> Gain/1
  Gain/1 -> Out1/1

== system EBike_Braking/Controller/If Action Subsystem11 ==
  In1 : Inport
  Action Port : ActionPort  ActionPortLabel=if(u1 > 0)
  Gain : Gain  Gain=0
  Out1 : Outport
  wires:
  Gain/1 -> Out1/1
  In1/1 -> Gain/1

== system EBike_Braking/Controller/If Action Subsystem12 ==
  In1 : Inport
  Action Port : ActionPort  ActionPortLabel=else
  Gain : Gain
  Out1 : Outport
  wires:
  Gain/1 -> Out1/1
  In1/1 -> Gain/1

== system EBike_Braking/Controller/If Action Subsystem8 ==
  In1 : Inport
  Action Port : ActionPort  ActionPortLabel=else
  Gain : Gain  Gain=0
  Out1 : Outport
  wires:
  Gain/1 -> Out1/1
  In1/1 -> Gain/1

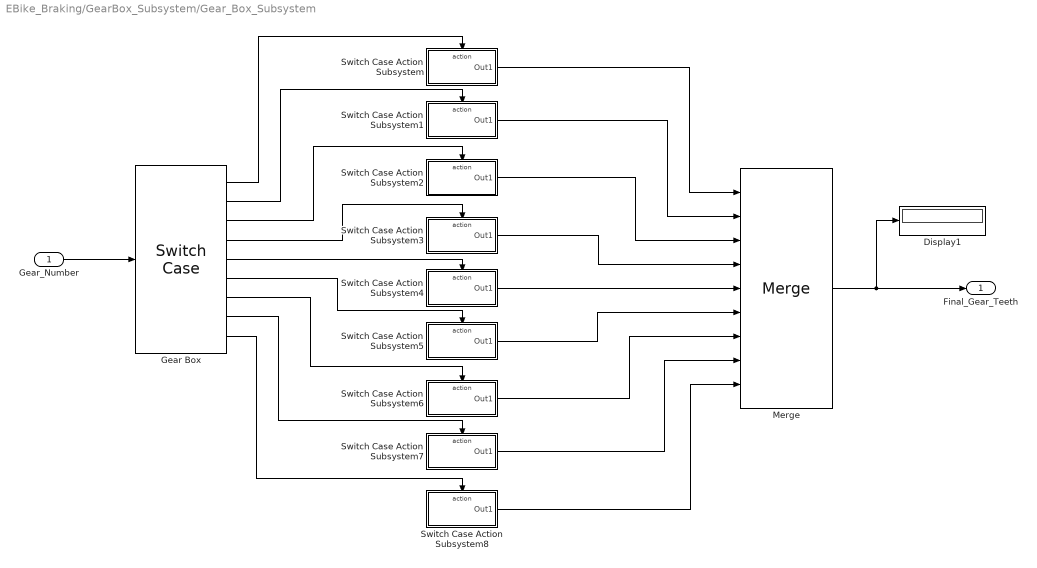
== system EBike_Braking/GearBox_Subsystem/Gear_Box_Subsystem ==
  Gear_Number : Inport
  Display1 : Display
  Gear Box : SwitchCase  CaseConditions={1,2,3,4,5,6,7,8,9}  ShowDefaultCase=off
  Merge : Merge  Inputs=9
  Switch Case Action Subsystem : Subsystem  TreatAsAtomicUnit=on
  Switch Case Action Subsystem1 : Subsystem  TreatAsAtomicUnit=on
  Switch Case Action Subsystem2 : Subsystem  TreatAsAtomicUnit=on
  Switch Case Action Subsystem3 : Subsystem  TreatAsAtomicUnit=on
  Switch Case Action Subsystem4 : Subsystem  TreatAsAtomicUnit=on
  Switch Case Action Subsystem5 : Subsystem  TreatAsAtomicUnit=on
  Switch Case Action Subsystem6 : Subsystem  TreatAsAtomicUnit=on
  Switch Case Action Subsystem7 : Subsystem  TreatAsAtomicUnit=on
  Switch Case Action Subsystem8 : Subsystem  TreatAsAtomicUnit=on
  Final_Gear_Teeth : Outport  VectorParamsAs1DForOutWhenUnconnected=off
  wires:
  Gear Box/5 -> Switch Case Action Subsystem4/Action
  Gear Box/2 -> Switch Case Action Subsystem1/Action
  Gear Box/4 -> Switch Case Action Subsystem3/Action
  Gear Box/9 -> Switch Case Action Subsystem8/Action
  Gear Box/7 -> Switch Case Action Subsystem6/Action
  Gear Box/6 -> Switch Case Action Subsystem5/Action
  Gear Box/3 -> Switch Case Action Subsystem2/Action
  Gear Box/1 -> Switch Case Action Subsystem/Action
  Merge/1 -> Display1/1, Final_Gear_Teeth/1
  Gear Box/8 -> Switch Case Action Subsystem7/Action
  Gear_Number/1 -> Gear Box/1
  Switch Case Action Subsystem8/1(Out1) -> Merge/9
  Switch Case Action Subsystem7/1(Out1) -> Merge/8
  Switch Case Action Subsystem6/1(Out1) -> Merge/7
  Switch Case Action Subsystem5/1(Out1) -> Merge/6
  Switch Case Action Subsystem4/1(Out1) -> Merge/5
  Switch Case Action Subsystem3/1(Out1) -> Merge/4
  Switch Case Action Subsystem2/1(Out1) -> Merge/3
  Switch Case Action Subsystem1/1(Out1) -> Merge/2
  Switch Case Action Subsystem/1(Out1) -> Merge/1

== system EBike_Braking/Motor_Subsystem/Magnetic_Flux_density_subsystem ==
  Ambient_temp_T : Inport
  Motor_torque_constant_at_Temp_T0 : Inport  Port=2
  Constant : Constant
  Product : Product
  Product1 : Product
  Reference_temp_T0 : Constant  Value=Ref_Temp
  Sum1 : Sum  Inputs=+-
  Sum2 : Sum
  Temperature_Coefficient : Constant  Value=Alpha_Magnet
  Motor_Torque_Constant_at_Temp_T : Outport  VectorParamsAs1DForOutWhenUnconnected=off
  wires:
  Motor_torque_constant_at_Temp_T0/1 -> Product1/1
  Product1/1 -> Motor_Torque_Constant_at_Temp_T/1
  Product/1 -> Sum2/2
  Constant/1 -> Sum2/1
  Sum2/1 -> Product1/2
  Temperature_Coefficient/1 -> Product/1
  Ambient_temp_T/1 -> Sum1/1
  Reference_temp_T0/1 -> Sum1/2
  Sum1/1 -> Product/2

== system EBike_Braking/Motor_Subsystem/Winding_resistance_Subsystem ==
  Resistance_at_Temp_T0 : Inport
  Ambient_temp_T : Inport  Port=2
  Constant : Constant
  Product : Product
  Product1 : Product
  Reference_temp_T0 : Constant  Value=Ref_Temp
  Resistance_Temperature_Coefficient : Constant  Value=alpha_Conductor
  Sum1 : Sum  Inputs=+-
  Sum2 : Sum
  Resistance_at_Temp_T : Outport  VectorParamsAs1DForOutWhenUnconnected=off
  wires:
  Sum1/1 -> Product/2
  Reference_temp_T0/1 -> Sum1/2
  Ambient_temp_T/1 -> Sum1/1
  Resistance_Temperature_Coefficient/1 -> Product/1
  Sum2/1 -> Product1/2
  Constant/1 -> Sum2/1
  Product/1 -> Sum2/2
  Product1/1 -> Resistance_at_Temp_T/1
  Resistance_at_Temp_T0/1 -> Product1/1

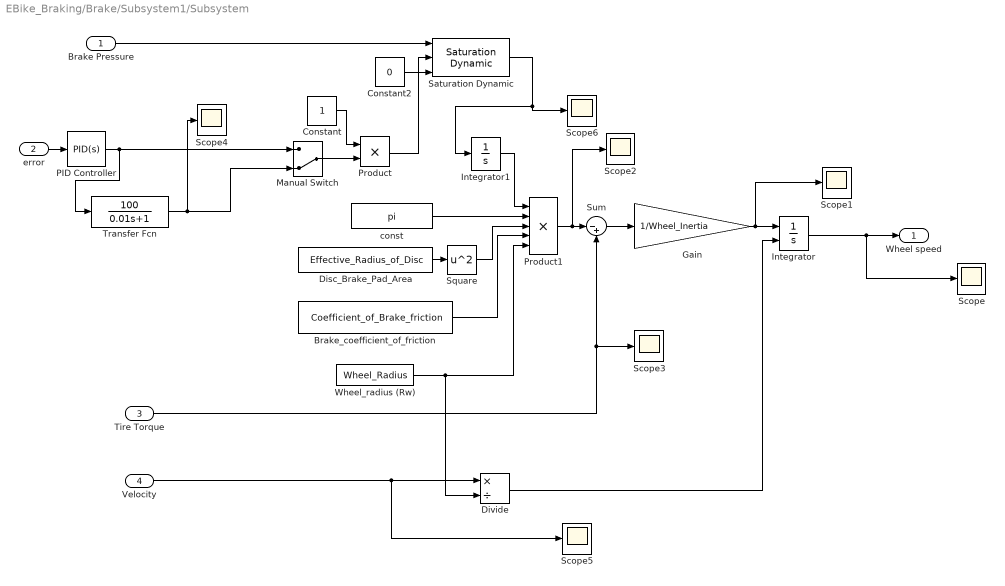
== system EBike_Braking/Brake/Subsystem1/Subsystem ==
  Brake Pressure : Inport
  "error " : Inport  Port=2
  Tire Torque : Inport  Port=3
  Velocity : Inport  Port=4
  Brake_coefficient_of_friction : Constant  Value=Coefficient_of_Brake_friction
  Constant : Constant
  Constant2 : Constant  Value=0
  Disc_Brake_Pad_Area : Constant  Value=Effective_Radius_of_Disc
  Divide : Product  Inputs=*/
  Gain : Gain  Gain=1/Wheel_Inertia
  Integrator : Integrator  InitialConditionSource=external  InitialCondition=V/Wheel_Radius  LimitOutput=on  UpperSaturationLimit=1000  LowerSaturationLimit=0
  Integrator1 : Integrator  UpperSaturationLimit=Braking_Pressure
  Manual Switch : ManualSwitch  CurrentSetting=0
  PID Controller : simulink/Continuous/PID Controller  Controller=PID  Form=Parallel  TimeDomain=Continuous-time  SampleTime=-1  IntegratorMethod=Forward Euler  FilterMethod=Forward Euler  ControllerParametersSource=internal  P=22  I=4  D=0.4  UseFilter=on  N=100  TunerSelectOption=Transfer Function Based (PID Tuner App)  InitialConditionSource=internal  InitialConditionForIntegrator=0  InitialConditionForFilter=0  DifferentiatorICPrevScaledInput=0  ExternalReset=none  TrackingMode=off  Kt=1  LimitOutput=off  UpperSaturationLimit=inf  LowerSaturationLimit=-inf  LinearizeAsGain=on  AntiWindupMode=none  Kb=1  POutMin=[]  POutMax=[]  IOutMin=[]  IOutMax=[]  DOutMin=[]  DOutMax=[]  NOutMin=[]  NOutMax=[]  SumOutMin=[]  SumOutMax=[]  SaturationOutMin=[]  SaturationOutMax=[]  PParamMin=[]  PParamMax=[]  IParamMin=[]  IParamMax=[]  DParamMin=[]  DParamMax=[]  NParamMin=[]  NParamMax=[]  KbParamMin=[]  KbParamMax=[]  KtParamMin=[]  KtParamMax=[]  KbOutMin=[]  KbOutMax=[]  KtOutMin=[]  KtOutMax=[]  IntegratorOutMin=[]  IntegratorOutMax=[]  FilterOutMin=[]  FilterOutMax=[]  SumI1OutMin=[]  SumI1OutMax=[]  SumI2OutMin=[]  SumI2OutMax=[]  SumI3OutMin=[]  SumI3OutMax=[]  SumI4OutMin=[]  SumI4OutMax=[]  SumDOutMin=[]  SumDOutMax=[]  DifferentiatorOutMin=[]  DifferentiatorOutMax=[]  FilterDiffOutCoefMin=[]  FilterDiffOutCoefMax=[]  ReciprocalOutMin=[]  ReciprocalOutMax=[]  SumDenOutMin=[]  SumDenOutMax=[]  SumNumOutMin=[]  SumNumOutMax=[]  DivideOutMin=[]  DivideOutMax=[]  IntegratorContinuousStateAttributes=''  IntegratorStateMustResolveToSignalObject=off  IntegratorRTWStateStorageClass=Auto  FilterContinuousStateAttributes=''  FilterStateMustResolveToSignalObject=off  FilterRTWStateStorageClass=Auto  ParallelPVariant=InternalParameters  IdealPVariant=Disabled  IVariant=InternalParameters  DVariant=InternalParameters  IntegratorVariant=Continuous  SatVariant=Disabled  AWVariant=Passthrough  PCopyVariant=Disabled  TRVariant=Disabled  FdbkBlocksVariant=Forward  IdealPFdbkVariant=Disabled  SatFdbkVariant=Disabled  DerivativeFilterVariant=ContFilter  NVariant=InternalParameters  NCopyVariant=Disabled  FilterICVariant=InternalICsFilter  IntegratorICVariant=InternalICs  ExternalResetVariant=Disabled  TRSumVariant=Passthrough  SumFdbkVariant=Disabled  SumVariant=Sum_PID
  Product : Product
  Product1 : Product  Inputs=5
  Saturation Dynamic : simulink/Discontinuities/Saturation Dynamic  OutMin=[]  OutMax=[]  OutDataTypeStr=Inherit: Same as second input  OutDataType=fixdt(1, 16)  OutScaling=2^-10  DoSatur=off
  Scope{,1..6} (7 alike) : Scope
  Square : Math  Operator=square  SaturateOnIntegerOverflow=on
  Sum : Sum  Inputs=|-+
  Transfer Fcn : TransferFcn  Numerator=[100]  Denominator=[0.01 1]
  "Wheel_radius (Rw) " : Constant  Value=Wheel_Radius
  "const " : Constant  Value=pi
  "Wheel speed " : Outport
  wires:
  "error "/1 -> PID Controller/1
  Constant/1 -> Product/1
  "const "/1 -> Product1/2
  Disc_Brake_Pad_Area/1 -> Square/1
  Square/1 -> Product1/3
  Brake_coefficient_of_friction/1 -> Product1/4
  Product1/1 -> Scope2/1, Sum/1
  Tire Torque/1 -> Scope3/1, Sum/2
  Sum/1 -> Gain/1
  Gain/1 -> Scope1/1, Integrator/1
  Manual Switch/1 -> Product/2
  PID Controller/1 -> Transfer Fcn/1, Manual Switch/1
  Integrator1/1 -> Product1/1
  Velocity/1 -> Scope5/1, Divide/1
  Divide/1 -> Integrator/2
  "Wheel_radius (Rw) "/1 -> Divide/2, Product1/5
  Integrator/1 -> "Wheel speed "/1, Scope/1
  Transfer Fcn/1 -> Scope4/1, Manual Switch/2
  Constant2/1 -> Saturation Dynamic/3
  Product/1 -> Saturation Dynamic/2
  Saturation Dynamic/1 -> Scope6/1, Integrator1/1
  Brake Pressure/1 -> Saturation Dynamic/1

== system EBike_Braking/GearBox_Subsystem/Gear_Box_Subsystem/Switch Case Action Subsystem ==
  Action Port : ActionPort  ActionPortLabel=case [ 1 ]:
  Constant : Constant  Value=34
  Out1 : Outport  VectorParamsAs1DForOutWhenUnconnected=off
  wires:
  Constant/1 -> Out1/1

== system EBike_Braking/GearBox_Subsystem/Gear_Box_Subsystem/Switch Case Action Subsystem1 ==
  Action Port : ActionPort  ActionPortLabel=case [ 2 ]:
  Constant : Constant  Value=30
  Out1 : Outport  VectorParamsAs1DForOutWhenUnconnected=off
  wires:
  Constant/1 -> Out1/1

== system EBike_Braking/GearBox_Subsystem/Gear_Box_Subsystem/Switch Case Action Subsystem2 ==
  Action Port : ActionPort  ActionPortLabel=case [ 3 ]:
  Constant : Constant  Value=26
  Out1 : Outport  VectorParamsAs1DForOutWhenUnconnected=off
  wires:
  Constant/1 -> Out1/1

== system EBike_Braking/GearBox_Subsystem/Gear_Box_Subsystem/Switch Case Action Subsystem3 ==
  Action Port : ActionPort  ActionPortLabel=case [ 4 ]:
  Constant : Constant  Value=23
  Out1 : Outport  VectorParamsAs1DForOutWhenUnconnected=off
  wires:
  Constant/1 -> Out1/1

== system EBike_Braking/GearBox_Subsystem/Gear_Box_Subsystem/Switch Case Action Subsystem4 ==
  Action Port : ActionPort  ActionPortLabel=case [ 5 ]:
  Constant : Constant  Value=20
  Out1 : Outport  VectorParamsAs1DForOutWhenUnconnected=off
  wires:
  Constant/1 -> Out1/1

== system EBike_Braking/GearBox_Subsystem/Gear_Box_Subsystem/Switch Case Action Subsystem5 ==
  Action Port : ActionPort  ActionPortLabel=case [ 6 ]:
  Constant : Constant  Value=17
  Out1 : Outport  VectorParamsAs1DForOutWhenUnconnected=off
  wires:
  Constant/1 -> Out1/1

== system EBike_Braking/GearBox_Subsystem/Gear_Box_Subsystem/Switch Case Action Subsystem6 ==
  Action Port : ActionPort  ActionPortLabel=case [ 7 ]:
  Constant : Constant  Value=15
  Out1 : Outport  VectorParamsAs1DForOutWhenUnconnected=off
  wires:
  Constant/1 -> Out1/1

== system EBike_Braking/GearBox_Subsystem/Gear_Box_Subsystem/Switch Case Action Subsystem7 ==
  Action Port : ActionPort  ActionPortLabel=case [ 8 ]:
  Constant : Constant  Value=13
  Out1 : Outport  VectorParamsAs1DForOutWhenUnconnected=off
  wires:
  Constant/1 -> Out1/1

== system EBike_Braking/GearBox_Subsystem/Gear_Box_Subsystem/Switch Case Action Subsystem8 ==
  Action Port : ActionPort  ActionPortLabel=case [ 9 ]:
  Constant : Constant  Value=11
  Out1 : Outport  VectorParamsAs1DForOutWhenUnconnected=off
  wires:
  Constant/1 -> Out1/1
